simulink subsystem "DCMotor"  (R2025a)
settings: Solver=VariableStepAuto  StartTime=0.0  StopTime=10.0  RelTol=1e-3
model mask{kw=0, L=0, R=0, km=0, J_motor=0, vis_friction_coef_motor=0}
settings Model: Creator=Глеб  LastModifiedBy=Глеб

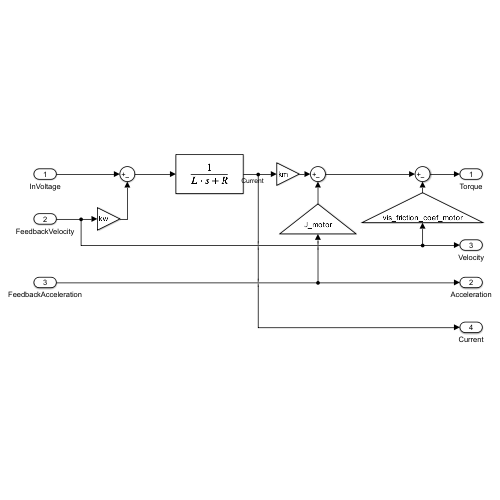
[thumbnail: Simulink's stored preview of the top-level diagram]
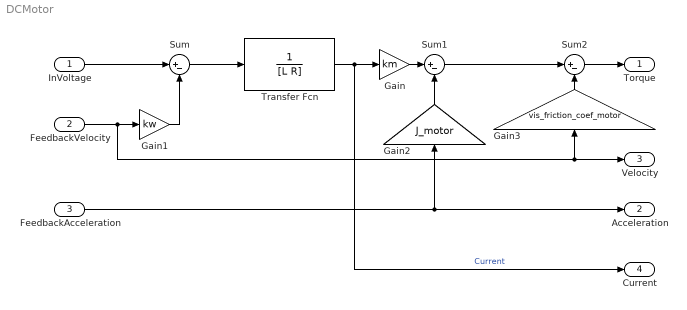
== system DCMotor ==
  InVoltage : Inport
  FeedbackVelocity : Inport  Port=2
  FeedbackAcceleration : Inport  Port=3
  Gain : Gain  Gain=km
  Gain1 : Gain  Gain=kw
  Gain2 : Gain  Gain=J_motor
  Gain3 : Gain  Gain=vis_friction_coef_motor
  Sum : Sum  Inputs=|+-
  Sum1 : Sum  Inputs=|+-
  Sum2 : Sum  Inputs=|+-
  Transfer Fcn : TransferFcn  Denominator=[L R]
  Torque : Outport
  Acceleration : Outport  Port=2
  Velocity : Outport  Port=3
  Current : Outport  Port=4
  wires:
  FeedbackVelocity/1 -> Velocity/1, Gain3/1, Gain1/1
  Gain3/1 -> Sum2/2
  Sum/1 -> Transfer Fcn/1
  Gain/1 -> Sum1/1
  Sum1/1 -> Sum2/1
  Gain2/1 -> Sum1/2
  Sum2/1 -> Torque/1
  InVoltage/1 -> Sum/1
  FeedbackAcceleration/1 -> Acceleration/1, Gain2/1
  Gain1/1 -> Sum/2
  Transfer Fcn/1 -> Current/1, Gain/1  "Current"
